simulink model "model_A3_2"  (R2024a)
settings: Solver=ode4  StartTime=0.0  StopTime=10  FixedStep=5e-3  MaxStep=1e-3  MinStep=1e-7  RelTol=1e-4  AbsTol=1e-3
values from neighbouring files (symbols this model uses):
  c = ..    [init_A3_2.m]
  D = ..    [init_A3_2.m]
  K = ..    [init_A3_2.m]
  L = ..    [init_A3_2.m]
  phi_0i = ..    [init_A3_2.m]
  phi_bar = 5/360*2*pi    (= 0.0872664625997)    [init_A3_2.m]
  q0 = ..    [init_A3_2.m]
  q1 = ..    [init_A3_2.m]
  T = ..    [init_A3_2.m]
settings Model: Creator=Schmidt  LastModifiedBy=Flipper
settings SolverCC: AutoScaleAbsTol=off  InitialStep=1e-3  AlgebraicLoopSolver=TrustRegion
settings DataIOCC: ReturnWorkspaceOutputs=off
settings OptimizationCC: LifeSpan=inf
settings DebuggingCC: UnconnectedInputMsg=warning  UnconnectedOutputMsg=warning  UnconnectedLineMsg=warning  SFExecutionAtInitializationDiag=none  ArithmeticOperatorsInVariantConditions=warning
settings ModelReferenceCC: EnableRefExpFcnMdlSchedulingChecks=on
settings SFSimCC: SimUseLocalCustomCode=off  CustomCodeUndefinedFunction=UseInterfaceOnly
settings RTWCC: RTWUseLocalCustomCode=off  GPUComputeCapability=3.5
settings CodeAppCC: StateflowObjectComments=on

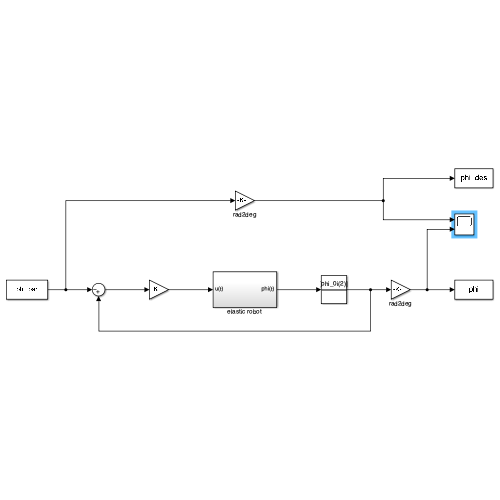
[thumbnail: Simulink's stored preview of the top-level diagram]
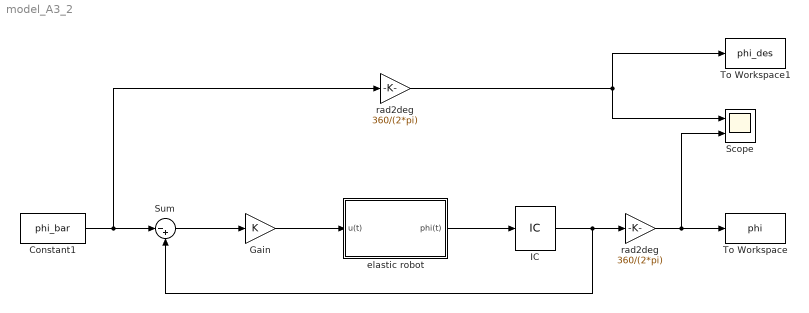
== system model_A3_2 ==
  Constant1 : Constant  Value=phi_bar
  Gain : Gain  Gain=K
  IC : InitialCondition  Value=phi_0i(2)
  Scope : Scope  NumInputPorts=2
  Sum : Sum  Inputs=|-+
  To Workspace : ToWorkspace  VariableName=phi  SaveFormat=Timeseries  SampleTime=-1
  To Workspace1 : ToWorkspace  VariableName=phi_des  SaveFormat=Timeseries  SampleTime=5e-3
  elastic robot : Subsystem
  rad2deg : Gain  Gain=360/(2*pi)
  "rad2deg " : Gain  Gain=360/(2*pi)
  wires:
  Constant1/1 -> Sum/1, rad2deg/1
  rad2deg/1 -> Scope/1, To Workspace1/1
  "rad2deg "/1 -> To Workspace/1, Scope/2
  IC/1 -> "rad2deg "/1, Sum/2
  Gain/1 -> elastic robot/1(u(t))
  Sum/1 -> Gain/1
  elastic robot/1(phi(t)) -> IC/1

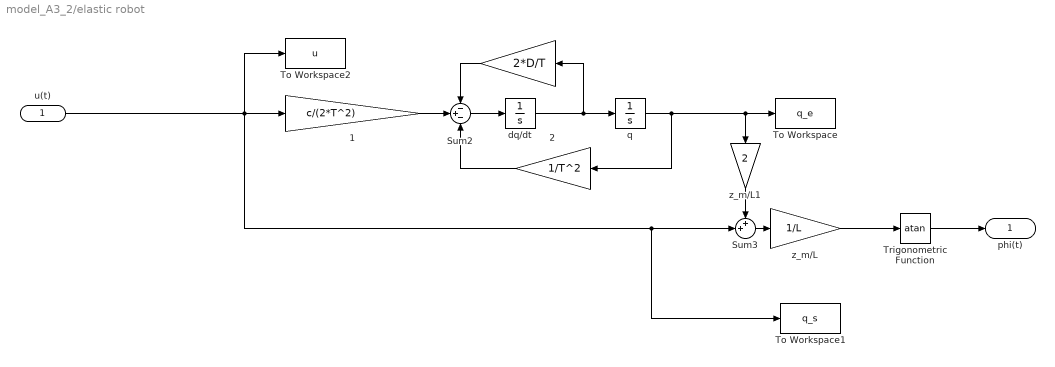
== system model_A3_2/elastic robot ==
  u(t) : Inport
  " " : Gain  Gain=2*D/T
  " 1" : Gain  Gain=c/(2*T^2)
  " 2" : Gain  Gain=1/T^2
  Sum2 : Sum  Inputs=-+-
  Sum3 : Sum  Inputs=++|
  To Workspace : ToWorkspace  VariableName=q_e  SaveFormat=Timeseries  SampleTime=-1
  To Workspace1 : ToWorkspace  VariableName=q_s  SaveFormat=Timeseries  SampleTime=-1
  To Workspace2 : ToWorkspace  VariableName=u  SaveFormat=Timeseries  SampleTime=-1
  Trigonometric Function : Trigonometry  Operator=atan
  dq/dt : Integrator  InitialCondition=q1
  q : Integrator  InitialCondition=q0
  z_m/L : Gain  Gain=1/L
  z_m/L1 : Gain  Gain=2
  phi(t) : Outport
  wires:
  Sum2/1 -> dq/dt/1
  z_m/L/1 -> Trigonometric Function/1
  " 2"/1 -> Sum2/3
  u(t)/1 -> To Workspace2/1, To Workspace1/1, Sum3/2, " 1"/1
  Sum3/1 -> z_m/L/1
  q/1 -> To Workspace/1, z_m/L1/1, " 2"/1
  " 1"/1 -> Sum2/2
  dq/dt/1 -> " "/1, q/1
  " "/1 -> Sum2/1
  Trigonometric Function/1 -> phi(t)/1
  z_m/L1/1 -> Sum3/1
